simulink model "example"  (Simulink 7.0)
settings: Solver=ode4  StartTime=0.0  StopTime=100  FixedStep=0.01  RelTol=1e-3
values from neighbouring files (symbols this model uses):
  TID = min('TI' == AFT(1:2))    [PAS_callback.m]    (also in PSTID_callback.m = [block '/TID'])
libraries: simulink x280
(part 1 of 15)
settings Model: Creator=jza  LastModifiedBy=jza

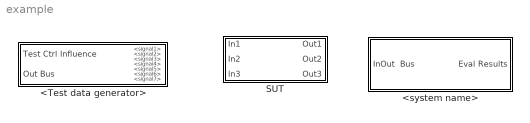
== system example ==
  <Test data generator> : Subsystem  mask{No=4, So=7, T=off}
      mask prompts: No "Number of Requirements"; So "Number of Signals"; T "Do you want to shut off the mask"
      mask StyleString: popup(1|2|3|4|5|6|7|8|9|10|11|12|13|14|15|16|17|18|19|20),popup(1|2|3|4|5|6|7|8|9|10|11|12|13|14|15|16|17|18|19|20),checkbox
      mask CallbackString: Test_D_Gen(gcb);|Test_D_Gen_S(gcb,-1);|shut_mask(gcb);
  <system name> : Subsystem  Description=Test evaluation system template. Create a new test evaluation system from this template.  mask{No=5, T=off}
      mask prompts: No "Number of Requirements"; T "Shut off the mask"
      mask StyleString: popup(1|2|3|4|5|6|7|8|9|10|11|12|13|14|15|16|17|18|19|20),checkbox
      mask CallbackString: system_name2(gcb);|shut_mask(gcb);
  SUT : Subsystem

== system example/<Test data generator> ==
  Test Ctrl Influence : Inport  OutDataType=sfix(16)  OutScaling=2^0
  Out Bus : Inport  Port=2  OutDataType=sfix(16)  OutScaling=2^0
  <Requirement name> : Subsystem
  <Requirement name>2 : Subsystem
  <Requirement name>3 : Subsystem
  <Requirement name>4 : Subsystem
  switch <signal1> : MultiPortSwitch  zeroidx=on
  switch <signal2> : MultiPortSwitch  zeroidx=on
  switch <signal3> : MultiPortSwitch  zeroidx=on
  switch <signal4> : MultiPortSwitch  zeroidx=on
  switch <signal5> : MultiPortSwitch  zeroidx=on
  switch <signal6> : MultiPortSwitch  zeroidx=on
  switch <signal7> : MultiPortSwitch  zeroidx=on
  <signal1> : Outport  OutDataType=sfix(16)  OutScaling=2^0
  <signal2> : Outport  Port=2  OutDataType=sfix(16)  OutScaling=2^0
  <signal3> : Outport  Port=3  OutDataType=sfix(16)  OutScaling=2^0
  <signal4> : Outport  Port=4  OutDataType=sfix(16)  OutScaling=2^0
  <signal5> : Outport  Port=5  OutDataType=sfix(16)  OutScaling=2^0
  <signal6> : Outport  Port=6  OutDataType=sfix(16)  OutScaling=2^0
  <signal7> : Outport  Port=7  OutDataType=sfix(16)  OutScaling=2^0
  wires:
  <Requirement name>/1(<signal1>) -> switch <signal1>/2
  switch <signal1>/1 -> <signal1>/1
  Out Bus/1 -> <Requirement name>/1(Out Bus), <Requirement name>2/1(Out Bus), <Requirement name>3/1(Out Bus), <Requirement name>4/1(Out Bus)
  Test Ctrl Influence/1 -> switch <signal1>/1, switch <signal2>/1, switch <signal3>/1, switch <signal4>/1, switch <signal5>/1, switch <signal6>/1, switch <signal7>/1
  <Requirement name>2/1(<signal1>) -> switch <signal1>/3
  <Requirement name>3/1(<signal1>) -> switch <signal1>/4
  <Requirement name>4/1(<signal1>) -> switch <signal1>/5
  switch <signal2>/1 -> <signal2>/1
  <Requirement name>/2(<signal2>) -> switch <signal2>/2
  <Requirement name>2/2(<signal2>) -> switch <signal2>/3
  <Requirement name>3/2(<signal2>) -> switch <signal2>/4
  <Requirement name>4/2(<signal2>) -> switch <signal2>/5
  switch <signal3>/1 -> <signal3>/1
  <Requirement name>/3(<signal3>) -> switch <signal3>/2
  <Requirement name>2/3(<signal3>) -> switch <signal3>/3
  <Requirement name>3/3(<signal3>) -> switch <signal3>/4
  <Requirement name>4/3(<signal3>) -> switch <signal3>/5
  switch <signal4>/1 -> <signal4>/1
  <Requirement name>/4(<signal4>) -> switch <signal4>/2
  <Requirement name>2/4(<signal4>) -> switch <signal4>/3
  <Requirement name>3/4(<signal4>) -> switch <signal4>/4
  <Requirement name>4/4(<signal4>) -> switch <signal4>/5
  switch <signal5>/1 -> <signal5>/1
  <Requirement name>/5(<signal5>) -> switch <signal5>/2
  <Requirement name>2/5(<signal5>) -> switch <signal5>/3
  <Requirement name>3/5(<signal5>) -> switch <signal5>/4
  <Requirement name>4/5(<signal5>) -> switch <signal5>/5
  switch <signal6>/1 -> <signal6>/1
  <Requirement name>/6(<signal6>) -> switch <signal6>/2
  <Requirement name>2/6(<signal6>) -> switch <signal6>/3
  <Requirement name>3/6(<signal6>) -> switch <signal6>/4
  <Requirement name>4/6(<signal6>) -> switch <signal6>/5
  switch <signal7>/1 -> <signal7>/1
  <Requirement name>/7(<signal7>) -> switch <signal7>/2
  <Requirement name>2/7(<signal7>) -> switch <signal7>/3
  <Requirement name>3/7(<signal7>) -> switch <signal7>/4
  <Requirement name>4/7(<signal7>) -> switch <signal7>/5

== system example/<system name> ==
  InOut  Bus : Inport  OutDataType=sfix(16)  OutScaling=2^0
  <Requirement name> : Subsystem  Description=Requirement template. Create a new requirement from this template.  mask{No=6}
      mask prompts: No "Number of single Validation Functions"
      mask StyleString: popup(1|2|3|4|5|6|7|8|9|10|11|12|13|14|15|16|17|18|19|20)
      mask CallbackString: ReqName_callback(gcb);
  <Requirement name>2 : Subsystem  Description=Requirement template. Create a new requirement from this template.  mask{No=1}
      mask prompts: No "Number of single Validation Functions"
      mask StyleString: popup(1|2|3|4|5|6|7|8|9|10|11|12|13|14|15|16|17|18|19|20)
      mask CallbackString: ReqName_callback(gcb);
  <Requirement name>3 : Subsystem  Description=Requirement template. Create a new requirement from this template.  mask{No=1}
      mask prompts: No "Number of single Validation Functions"
      mask StyleString: popup(1|2|3|4|5|6|7|8|9|10|11|12|13|14|15|16|17|18|19|20)
      mask CallbackString: ReqName_callback(gcb);
  <Requirement name>4 : Subsystem  Description=Requirement template. Create a new requirement from this template.  mask{No=1}
      mask prompts: No "Number of single Validation Functions"
      mask StyleString: popup(1|2|3|4|5|6|7|8|9|10|11|12|13|14|15|16|17|18|19|20)
      mask CallbackString: ReqName_callback(gcb);
  <Requirement name>5 : Subsystem  Description=Requirement template. Create a new requirement from this template.  mask{No=1}
      mask prompts: No "Number of single Validation Functions"
      mask StyleString: popup(1|2|3|4|5|6|7|8|9|10|11|12|13|14|15|16|17|18|19|20)
      mask CallbackString: ReqName_callback(gcb);
  Arbitration : Subsystem
  Bus Creator : BusCreator  Inputs=5
  Bus Creator1 : BusCreator  Inputs=2
  Bus Creator4 : BusCreator  Inputs=10
  Bus Selector : BusSelector  OutputSignals=signal1.signal1.signal1,signal2.signal1.signal1,signal3.signal1.signal1,signal4.signal1.signal1,signal5.signal1.signal1,signal.signal2.signal1,signal.signal3.signal1,signal.signal4.signal1,signal.signal5.signal1,signal.signal6.signal1
  Signal Conversion : SignalConversion  ConversionOutput=Bus copy
  Terminator : Terminator
  Eval Results : Outport  OutDataType=sfix(16)  OutScaling=2^0
  wires:
  Bus Creator1/1 -> Eval Results/1
  Bus Creator4/1 -> Bus Creator1/2
  Signal Conversion/1 -> <Requirement name>/1(InOut Bus), <Requirement name>2/1(InOut Bus), <Requirement name>3/1(InOut Bus), <Requirement name>4/1(InOut Bus), <Requirement name>5/1(InOut Bus)
  Bus Creator/1 -> Terminator/1, Bus Selector/1
  InOut  Bus/1 -> Signal Conversion/1
  <Requirement name>/1(Test Info) -> Bus Creator/1
  Arbitration/1(Out1) -> Bus Creator1/1
  Bus Selector/1 -> Arbitration/1(In1), Bus Creator4/1  "<signal1>"
  <Requirement name>2/1(Test Info) -> Bus Creator/2
  Bus Selector/2 -> Bus Creator4/2, Arbitration/2(In2)  "<signal1>"
  <Requirement name>3/1(Test Info) -> Bus Creator/3
  Bus Selector/3 -> Bus Creator4/3, Arbitration/3(In3)  "<signal1>"
  <Requirement name>4/1(Test Info) -> Bus Creator/4
  Bus Selector/4 -> Bus Creator4/4, Arbitration/4(In4)  "<signal1>"
  <Requirement name>5/1(Test Info) -> Bus Creator/5
  Bus Selector/5 -> Bus Creator4/5, Arbitration/5(In5)  "<signal1>"
  Bus Selector/6 -> Arbitration/6(In6), Bus Creator4/6  "<signal1>"
  Bus Selector/7 -> Arbitration/7(In7), Bus Creator4/7  "<signal1>"
  Bus Selector/8 -> Arbitration/8(In8), Bus Creator4/8  "<signal1>"
  Bus Selector/9 -> Arbitration/9(In9), Bus Creator4/9  "<signal1>"
  Bus Selector/10 -> Arbitration/10(In10), Bus Creator4/10  "<signal1>"

== system example/SUT ==
  In1 : Inport  OutDataType=sfix(16)  OutScaling=2^0
  In2 : Inport  Port=2  OutDataType=sfix(16)  OutScaling=2^0
  In3 : Inport  Port=3  OutDataType=sfix(16)  OutScaling=2^0
  Out1 : Outport  OutDataType=sfix(16)  OutScaling=2^0
  Out2 : Outport  Port=2  OutDataType=sfix(16)  OutScaling=2^0
  Out3 : Outport  Port=3  OutDataType=sfix(16)  OutScaling=2^0
  wires:
  In1/1 -> Out1/1
  In2/1 -> Out2/1
  In3/1 -> Out3/1

== system example/<Test data generator>/<Requirement name> ==
  Out Bus : Inport  OutDataType=sfix(16)  OutScaling=2^0
  <Preconditions name> : Subsystem
  Initialisation & Stabilisation : Subsystem
  Sequencing of test data in time due to Preconditions : Stateflow chart
  switch <signal1> : MultiPortSwitch  Inputs=2
  switch <signal2> : MultiPortSwitch  Inputs=2
  switch <signal3> : MultiPortSwitch  Inputs=2
  switch <signal4> : MultiPortSwitch  Inputs=2
  switch <signal5> : MultiPortSwitch  Inputs=2
  switch <signal6> : MultiPortSwitch  Inputs=2
  switch <signal7> : MultiPortSwitch  Inputs=2
  <signal1> : Outport  OutDataType=sfix(16)  OutScaling=2^0
  <signal2> : Outport  Port=2  OutDataType=sfix(16)  OutScaling=2^0
  <signal3> : Outport  Port=3  OutDataType=sfix(16)  OutScaling=2^0
  <signal4> : Outport  Port=4  OutDataType=sfix(16)  OutScaling=2^0
  <signal5> : Outport  Port=5  OutDataType=sfix(16)  OutScaling=2^0
  <signal6> : Outport  Port=6  OutDataType=sfix(16)  OutScaling=2^0
  <signal7> : Outport  Port=7  OutDataType=sfix(16)  OutScaling=2^0
  wires:
  Out Bus/1 -> <Preconditions name>/1(Out Bus)
  switch <signal1>/1 -> <signal1>/1
  <Preconditions name>/1(Activate) -> Sequencing of test data in time due to Preconditions/1(Activate)
  Sequencing of test data in time due to Preconditions/1(TDPre) -> switch <signal1>/1, switch <signal2>/1, switch <signal3>/1, switch <signal4>/1, switch <signal5>/1, switch <signal6>/1, switch <signal7>/1
  <Preconditions name>/2(<signal1>) -> switch <signal1>/2
  Initialisation & Stabilisation/1(<signal1>) -> switch <signal1>/3, switch <signal2>/3, switch <signal3>/3, switch <signal4>/3, switch <signal5>/3, switch <signal6>/3, switch <signal7>/3
  switch <signal2>/1 -> <signal2>/1
  <Preconditions name>/3(<signal2>) -> switch <signal2>/2
  switch <signal3>/1 -> <signal3>/1
  <Preconditions name>/4(<signal3>) -> switch <signal3>/2
  switch <signal4>/1 -> <signal4>/1
  <Preconditions name>/5(<signal4>) -> switch <signal4>/2
  switch <signal5>/1 -> <signal5>/1
  <Preconditions name>/6(<signal5>) -> switch <signal5>/2
  switch <signal6>/1 -> <signal6>/1
  <Preconditions name>/7(<signal6>) -> switch <signal6>/2
  switch <signal7>/1 -> <signal7>/1
  <Preconditions name>/8(<signal7>) -> switch <signal7>/2

== system example/<Test data generator>/<Requirement name>2 ==
  Out Bus : Inport  OutDataType=sfix(16)  OutScaling=2^0
  <Preconditions name> : Subsystem
  Initialisation & Stabilisation : Subsystem
  Sequencing of test data in time due to Preconditions : Stateflow chart
  switch <signal1> : MultiPortSwitch  Inputs=2
  switch <signal2> : MultiPortSwitch  Inputs=2
  switch <signal3> : MultiPortSwitch  Inputs=2
  switch <signal4> : MultiPortSwitch  Inputs=2
  switch <signal5> : MultiPortSwitch  Inputs=2
  switch <signal6> : MultiPortSwitch  Inputs=2
  switch <signal7> : MultiPortSwitch  Inputs=2
  <signal1> : Outport  OutDataType=sfix(16)  OutScaling=2^0
  <signal2> : Outport  Port=2  OutDataType=sfix(16)  OutScaling=2^0
  <signal3> : Outport  Port=3  OutDataType=sfix(16)  OutScaling=2^0
  <signal4> : Outport  Port=4  OutDataType=sfix(16)  OutScaling=2^0
  <signal5> : Outport  Port=5  OutDataType=sfix(16)  OutScaling=2^0
  <signal6> : Outport  Port=6  OutDataType=sfix(16)  OutScaling=2^0
  <signal7> : Outport  Port=7  OutDataType=sfix(16)  OutScaling=2^0
  wires:
  Initialisation & Stabilisation/1(<signal1>) -> switch <signal1>/3, switch <signal2>/3, switch <signal3>/3, switch <signal4>/3, switch <signal5>/3, switch <signal6>/3, switch <signal7>/3
  <Preconditions name>/2(<signal1>) -> switch <signal1>/2
  Sequencing of test data in time due to Preconditions/1(TDPre) -> switch <signal1>/1, switch <signal2>/1, switch <signal3>/1, switch <signal4>/1, switch <signal5>/1, switch <signal6>/1, switch <signal7>/1
  <Preconditions name>/1(Activate) -> Sequencing of test data in time due to Preconditions/1(Activate)
  switch <signal1>/1 -> <signal1>/1
  Out Bus/1 -> <Preconditions name>/1(Out Bus)
  switch <signal2>/1 -> <signal2>/1
  <Preconditions name>/3(<signal2>) -> switch <signal2>/2
  switch <signal3>/1 -> <signal3>/1
  <Preconditions name>/4(<signal3>) -> switch <signal3>/2
  switch <signal4>/1 -> <signal4>/1
  <Preconditions name>/5(<signal4>) -> switch <signal4>/2
  switch <signal5>/1 -> <signal5>/1
  <Preconditions name>/6(<signal5>) -> switch <signal5>/2
  switch <signal6>/1 -> <signal6>/1
  <Preconditions name>/7(<signal6>) -> switch <signal6>/2
  switch <signal7>/1 -> <signal7>/1
  <Preconditions name>/8(<signal7>) -> switch <signal7>/2

== system example/<Test data generator>/<Requirement name>3 ==
  Out Bus : Inport  OutDataType=sfix(16)  OutScaling=2^0
  <Preconditions name> : Subsystem
  Initialisation & Stabilisation : Subsystem
  Sequencing of test data in time due to Preconditions : Stateflow chart
  switch <signal1> : MultiPortSwitch  Inputs=2
  switch <signal2> : MultiPortSwitch  Inputs=2
  switch <signal3> : MultiPortSwitch  Inputs=2
  switch <signal4> : MultiPortSwitch  Inputs=2
  switch <signal5> : MultiPortSwitch  Inputs=2
  switch <signal6> : MultiPortSwitch  Inputs=2
  switch <signal7> : MultiPortSwitch  Inputs=2
  <signal1> : Outport  OutDataType=sfix(16)  OutScaling=2^0
  <signal2> : Outport  Port=2  OutDataType=sfix(16)  OutScaling=2^0
  <signal3> : Outport  Port=3  OutDataType=sfix(16)  OutScaling=2^0
  <signal4> : Outport  Port=4  OutDataType=sfix(16)  OutScaling=2^0
  <signal5> : Outport  Port=5  OutDataType=sfix(16)  OutScaling=2^0
  <signal6> : Outport  Port=6  OutDataType=sfix(16)  OutScaling=2^0
  <signal7> : Outport  Port=7  OutDataType=sfix(16)  OutScaling=2^0
  wires:
  Out Bus/1 -> <Preconditions name>/1(Out Bus)
  switch <signal1>/1 -> <signal1>/1
  <Preconditions name>/1(Activate) -> Sequencing of test data in time due to Preconditions/1(Activate)
  Sequencing of test data in time due to Preconditions/1(TDPre) -> switch <signal1>/1, switch <signal2>/1, switch <signal3>/1, switch <signal4>/1, switch <signal5>/1, switch <signal6>/1, switch <signal7>/1
  <Preconditions name>/2(<signal1>) -> switch <signal1>/2
  Initialisation & Stabilisation/1(<signal1>) -> switch <signal1>/3, switch <signal2>/3, switch <signal3>/3, switch <signal4>/3, switch <signal5>/3, switch <signal6>/3, switch <signal7>/3
  switch <signal2>/1 -> <signal2>/1
  <Preconditions name>/3(<signal2>) -> switch <signal2>/2
  switch <signal3>/1 -> <signal3>/1
  <Preconditions name>/4(<signal3>) -> switch <signal3>/2
  switch <signal4>/1 -> <signal4>/1
  <Preconditions name>/5(<signal4>) -> switch <signal4>/2
  switch <signal5>/1 -> <signal5>/1
  <Preconditions name>/6(<signal5>) -> switch <signal5>/2
  switch <signal6>/1 -> <signal6>/1
  <Preconditions name>/7(<signal6>) -> switch <signal6>/2
  switch <signal7>/1 -> <signal7>/1
  <Preconditions name>/8(<signal7>) -> switch <signal7>/2

== system example/<Test data generator>/<Requirement name>4 ==
  Out Bus : Inport  OutDataType=sfix(16)  OutScaling=2^0
  <Preconditions name> : Subsystem
  Initialisation & Stabilisation : Subsystem
  Sequencing of test data in time due to Preconditions : Stateflow chart
  switch <signal1> : MultiPortSwitch  Inputs=2
  switch <signal2> : MultiPortSwitch  Inputs=2
  switch <signal3> : MultiPortSwitch  Inputs=2
  switch <signal4> : MultiPortSwitch  Inputs=2
  switch <signal5> : MultiPortSwitch  Inputs=2
  switch <signal6> : MultiPortSwitch  Inputs=2
  switch <signal7> : MultiPortSwitch  Inputs=2
  <signal1> : Outport  OutDataType=sfix(16)  OutScaling=2^0
  <signal2> : Outport  Port=2  OutDataType=sfix(16)  OutScaling=2^0
  <signal3> : Outport  Port=3  OutDataType=sfix(16)  OutScaling=2^0
  <signal4> : Outport  Port=4  OutDataType=sfix(16)  OutScaling=2^0
  <signal5> : Outport  Port=5  OutDataType=sfix(16)  OutScaling=2^0
  <signal6> : Outport  Port=6  OutDataType=sfix(16)  OutScaling=2^0
  <signal7> : Outport  Port=7  OutDataType=sfix(16)  OutScaling=2^0
  wires:
  Initialisation & Stabilisation/1(<signal1>) -> switch <signal1>/3, switch <signal2>/3, switch <signal3>/3, switch <signal4>/3, switch <signal5>/3, switch <signal6>/3, switch <signal7>/3
  <Preconditions name>/2(<signal1>) -> switch <signal1>/2
  Sequencing of test data in time due to Preconditions/1(TDPre) -> switch <signal1>/1, switch <signal2>/1, switch <signal3>/1, switch <signal4>/1, switch <signal5>/1, switch <signal6>/1, switch <signal7>/1
  <Preconditions name>/1(Activate) -> Sequencing of test data in time due to Preconditions/1(Activate)
  switch <signal1>/1 -> <signal1>/1
  Out Bus/1 -> <Preconditions name>/1(Out Bus)
  switch <signal2>/1 -> <signal2>/1
  <Preconditions name>/3(<signal2>) -> switch <signal2>/2
  switch <signal3>/1 -> <signal3>/1
  <Preconditions name>/4(<signal3>) -> switch <signal3>/2
  switch <signal4>/1 -> <signal4>/1
  <Preconditions name>/5(<signal4>) -> switch <signal4>/2
  switch <signal5>/1 -> <signal5>/1
  <Preconditions name>/6(<signal5>) -> switch <signal5>/2
  switch <signal6>/1 -> <signal6>/1
  <Preconditions name>/7(<signal6>) -> switch <signal6>/2
  switch <signal7>/1 -> <signal7>/1
  <Preconditions name>/8(<signal7>) -> switch <signal7>/2

== system example/<system name>/<Requirement name> ==
  InOut Bus : Inport  OutDataType=sfix(16)  OutScaling=2^0
  <Assertions name> : Subsystem  Description=Assertions template. Create a new assertions block from this template.
  <Assertions name>2 : Subsystem  Description=Assertions template. Create a new assertions block from this template.
  <Assertions name>3 : Subsystem  Description=Assertions template. Create a new assertions block from this template.
  <Assertions name>4 : Subsystem  Description=Assertions template. Create a new assertions block from this template.
  <Assertions name>5 : Subsystem  Description=Assertions template. Create a new assertions block from this template.
  <Assertions name>6 : Subsystem  Description=Assertions template. Create a new assertions block from this template.
  <Preconditions name> : Subsystem  Description=Preconditions template. Create new preconditions blocks using this template.
  <Preconditions name>2 : Subsystem  Description=Preconditions template. Create new preconditions blocks using this template.
  <Preconditions name>3 : Subsystem  Description=Preconditions template. Create new preconditions blocks using this template.
  <Preconditions name>4 : Subsystem  Description=Preconditions template. Create new preconditions blocks using this template.
  <Preconditions name>5 : Subsystem  Description=Preconditions template. Create new preconditions blocks using this template.
  <Preconditions name>6 : Subsystem  Description=Preconditions template. Create new preconditions blocks using this template.
  Bus Creator : BusCreator  Inputs=6
  Test Info : Outport  OutDataType=sfix(16)  OutScaling=2^0
  wires:
  <Preconditions name>/1(Activate) -> <Assertions name>/1(Precond)
  Bus Creator/1 -> Test Info/1
  <Assertions name>/1(VF info) -> Bus Creator/1
  InOut Bus/1 -> <Preconditions name>/1(InOut Bus), <Assertions name>/2(InOut Bus), <Assertions name>2/2(InOut Bus), <Preconditions name>2/1(InOut Bus), <Assertions name>3/2(InOut Bus), <Preconditions name>3/1(InOut Bus), <Assertions name>4/2(InOut Bus), <Preconditions name>4/1(InOut Bus), <Assertions name>5/2(InOut Bus), <Preconditions name>5/1(InOut Bus), <Assertions name>6/2(InOut Bus), <Preconditions name>6/1(InOut Bus)
  <Preconditions name>2/1(Activate) -> <Assertions name>2/1(Precond)
  <Assertions name>2/1(VF info) -> Bus Creator/2
  <Preconditions name>3/1(Activate) -> <Assertions name>3/1(Precond)
  <Assertions name>3/1(VF info) -> Bus Creator/3
  <Preconditions name>4/1(Activate) -> <Assertions name>4/1(Precond)
  <Assertions name>4/1(VF info) -> Bus Creator/4
  <Preconditions name>5/1(Activate) -> <Assertions name>5/1(Precond)
  <Assertions name>5/1(VF info) -> Bus Creator/5
  <Preconditions name>6/1(Activate) -> <Assertions name>6/1(Precond)
  <Assertions name>6/1(VF info) -> Bus Creator/6

== system example/<system name>/<Requirement name>2 ==
  InOut Bus : Inport  OutDataType=sfix(16)  OutScaling=2^0
  <Assertions name> : Subsystem  Description=Assertions template. Create a new assertions block from this template.
  <Preconditions name> : Subsystem  Description=Preconditions template. Create new preconditions blocks using this template.
  Bus Creator : BusCreator  Inputs=1
  Test Info : Outport  OutDataType=sfix(16)  OutScaling=2^0
  wires:
  <Preconditions name>/1(Activate) -> <Assertions name>/1(Precond)
  Bus Creator/1 -> Test Info/1
  <Assertions name>/1(VF info) -> Bus Creator/1
  InOut Bus/1 -> <Preconditions name>/1(InOut Bus), <Assertions name>/2(InOut Bus)

== system example/<system name>/<Requirement name>3 ==
  InOut Bus : Inport  OutDataType=sfix(16)  OutScaling=2^0
  <Assertions name> : Subsystem  Description=Assertions template. Create a new assertions block from this template.
  <Preconditions name> : Subsystem  Description=Preconditions template. Create new preconditions blocks using this template.
  Bus Creator : BusCreator  Inputs=1
  Test Info : Outport  OutDataType=sfix(16)  OutScaling=2^0
  wires:
  <Preconditions name>/1(Activate) -> <Assertions name>/1(Precond)
  Bus Creator/1 -> Test Info/1
  <Assertions name>/1(VF info) -> Bus Creator/1
  InOut Bus/1 -> <Preconditions name>/1(InOut Bus), <Assertions name>/2(InOut Bus)

== system example/<system name>/<Requirement name>4 ==
  InOut Bus : Inport  OutDataType=sfix(16)  OutScaling=2^0
  <Assertions name> : Subsystem  Description=Assertions template. Create a new assertions block from this template.
  <Preconditions name> : Subsystem  Description=Preconditions template. Create new preconditions blocks using this template.
  Bus Creator : BusCreator  Inputs=1
  Test Info : Outport  OutDataType=sfix(16)  OutScaling=2^0
  wires:
  <Preconditions name>/1(Activate) -> <Assertions name>/1(Precond)
  Bus Creator/1 -> Test Info/1
  <Assertions name>/1(VF info) -> Bus Creator/1
  InOut Bus/1 -> <Preconditions name>/1(InOut Bus), <Assertions name>/2(InOut Bus)

== system example/<system name>/<Requirement name>5 ==
  InOut Bus : Inport  OutDataType=sfix(16)  OutScaling=2^0
  <Assertions name> : Subsystem  Description=Assertions template. Create a new assertions block from this template.
  <Preconditions name> : Subsystem  Description=Preconditions template. Create new preconditions blocks using this template.
  Bus Creator : BusCreator  Inputs=1
  Test Info : Outport  OutDataType=sfix(16)  OutScaling=2^0
  wires:
  <Preconditions name>/1(Activate) -> <Assertions name>/1(Precond)
  Bus Creator/1 -> Test Info/1
  <Assertions name>/1(VF info) -> Bus Creator/1
  InOut Bus/1 -> <Preconditions name>/1(InOut Bus), <Assertions name>/2(InOut Bus)

== system example/<system name>/Arbitration ==
  In1 : Inport  OutDataType=sfix(16)  OutScaling=2^0
  In2 : Inport  Port=2  OutDataType=sfix(16)  OutScaling=2^0
  In3 : Inport  Port=3  OutDataType=sfix(16)  OutScaling=2^0
  In4 : Inport  Port=4  OutDataType=sfix(16)  OutScaling=2^0
  In5 : Inport  Port=5  OutDataType=sfix(16)  OutScaling=2^0
  In6 : Inport  Port=6  OutDataType=sfix(16)  OutScaling=2^0
  In7 : Inport  Port=7  OutDataType=sfix(16)  OutScaling=2^0
  In8 : Inport  Port=8  OutDataType=sfix(16)  OutScaling=2^0
  In9 : Inport  Port=9  OutDataType=sfix(16)  OutScaling=2^0
  In10 : Inport  Port=10  OutDataType=sfix(16)  OutScaling=2^0
  Collect Verdicts : MinMax  Inputs=11  OutDataType=sfix(16)  OutScaling=2^0
  Memory : Memory  Orientation=left  X0=2
  Out1 : Outport  OutDataType=sfix(16)  OutScaling=2^0
  wires:
  In1/1 -> Collect Verdicts/1
  Collect Verdicts/1 -> Out1/1, Memory/1
  In2/1 -> Collect Verdicts/2
  In3/1 -> Collect Verdicts/3
  In4/1 -> Collect Verdicts/4
  In5/1 -> Collect Verdicts/5
  In6/1 -> Collect Verdicts/6
  In7/1 -> Collect Verdicts/7
  In8/1 -> Collect Verdicts/8
  In9/1 -> Collect Verdicts/9
  Memory/1 -> Collect Verdicts/11
  In10/1 -> Collect Verdicts/10

== system example/<Test data generator>/<Requirement name>/<Preconditions name> ==
  Out Bus : Inport  OutDataType=sfix(16)  OutScaling=2^0
  <Check> : Subsystem
  Feature generation : Subsystem  TreatAsAtomicUnit=on  mask{Param=0}
      mask prompts: Param "Mask Parameter 1:"
  Feature generation2 : Subsystem  TreatAsAtomicUnit=on  mask{Param=0}
      mask prompts: Param "Mask Parameter 1:"
  Feature generation3 : Subsystem  TreatAsAtomicUnit=on  mask{Param=0}
      mask prompts: Param "Mask Parameter 1:"
  Feature generation4 : Subsystem  TreatAsAtomicUnit=on  mask{Param=0}
      mask prompts: Param "Mask Parameter 1:"
  Feature generation5 : Subsystem  TreatAsAtomicUnit=on  mask{Param=0}
      mask prompts: Param "Mask Parameter 1:"
  Feature generation6 : Subsystem  TreatAsAtomicUnit=on  mask{Param=0}
      mask prompts: Param "Mask Parameter 1:"
  Feature generation7 : Subsystem  TreatAsAtomicUnit=on  mask{Param=0}
      mask prompts: Param "Mask Parameter 1:"
  Activate : Outport  OutDataType=sfix(16)  OutScaling=2^0
  <signal1> : Outport  Port=2  OutDataType=sfix(16)  OutScaling=2^0
  <signal2> : Outport  Port=3  OutDataType=sfix(16)  OutScaling=2^0
  <signal3> : Outport  Port=4  OutDataType=sfix(16)  OutScaling=2^0
  <signal4> : Outport  Port=5  OutDataType=sfix(16)  OutScaling=2^0
  <signal5> : Outport  Port=6  OutDataType=sfix(16)  OutScaling=2^0
  <signal6> : Outport  Port=7  OutDataType=sfix(16)  OutScaling=2^0
  <signal7> : Outport  Port=8  OutDataType=sfix(16)  OutScaling=2^0
  wires:
  Out Bus/1 -> <Check>/1(Out Bus)
  Feature generation/1(<signal1>) -> <signal1>/1
  <Check>/1(A) -> Activate/1
  Feature generation2/1(<signal1>) -> <signal2>/1
  Feature generation3/1(<signal1>) -> <signal3>/1
  Feature generation4/1(<signal1>) -> <signal4>/1
  Feature generation5/1(<signal1>) -> <signal5>/1
  Feature generation6/1(<signal1>) -> <signal6>/1
  Feature generation7/1(<signal1>) -> <signal7>/1

== system example/<Test data generator>/<Requirement name>/Initialisation & Stabilisation ==
  <Feature generation> : Subsystem  TreatAsAtomicUnit=on  mask{Param=0}
      mask prompts: Param "Mask Parameter 1:"
  <signal1> : Outport  OutDataType=sfix(16)  OutScaling=2^0
  wires:
  <Feature generation>/1(<signal1>) -> <signal1>/1

== system example/<Test data generator>/<Requirement name>2/<Preconditions name> ==
  Out Bus : Inport  OutDataType=sfix(16)  OutScaling=2^0
  <Check> : Subsystem
  Feature generation : Subsystem  TreatAsAtomicUnit=on  mask{Param=0}
      mask prompts: Param "Mask Parameter 1:"
  Feature generation2 : Subsystem  TreatAsAtomicUnit=on  mask{Param=0}
      mask prompts: Param "Mask Parameter 1:"
  Feature generation3 : Subsystem  TreatAsAtomicUnit=on  mask{Param=0}
      mask prompts: Param "Mask Parameter 1:"
  Feature generation4 : Subsystem  TreatAsAtomicUnit=on  mask{Param=0}
      mask prompts: Param "Mask Parameter 1:"
  Feature generation5 : Subsystem  TreatAsAtomicUnit=on  mask{Param=0}
      mask prompts: Param "Mask Parameter 1:"
  Feature generation6 : Subsystem  TreatAsAtomicUnit=on  mask{Param=0}
      mask prompts: Param "Mask Parameter 1:"
  Feature generation7 : Subsystem  TreatAsAtomicUnit=on  mask{Param=0}
      mask prompts: Param "Mask Parameter 1:"
  Activate : Outport  OutDataType=sfix(16)  OutScaling=2^0
  <signal1> : Outport  Port=2  OutDataType=sfix(16)  OutScaling=2^0
  <signal2> : Outport  Port=3  OutDataType=sfix(16)  OutScaling=2^0
  <signal3> : Outport  Port=4  OutDataType=sfix(16)  OutScaling=2^0
  <signal4> : Outport  Port=5  OutDataType=sfix(16)  OutScaling=2^0
  <signal5> : Outport  Port=6  OutDataType=sfix(16)  OutScaling=2^0
  <signal6> : Outport  Port=7  OutDataType=sfix(16)  OutScaling=2^0
  <signal7> : Outport  Port=8  OutDataType=sfix(16)  OutScaling=2^0
  wires:
  <Check>/1(A) -> Activate/1
  Feature generation/1(<signal1>) -> <signal1>/1
  Out Bus/1 -> <Check>/1(Out Bus)
  Feature generation2/1(<signal1>) -> <signal2>/1
  Feature generation3/1(<signal1>) -> <signal3>/1
  Feature generation4/1(<signal1>) -> <signal4>/1
  Feature generation5/1(<signal1>) -> <signal5>/1
  Feature generation6/1(<signal1>) -> <signal6>/1
  Feature generation7/1(<signal1>) -> <signal7>/1

== system example/<Test data generator>/<Requirement name>2/Initialisation & Stabilisation ==
  <Feature generation> : Subsystem  TreatAsAtomicUnit=on  mask{Param=0}
      mask prompts: Param "Mask Parameter 1:"
  <signal1> : Outport  OutDataType=sfix(16)  OutScaling=2^0
  wires:
  <Feature generation>/1(<signal1>) -> <signal1>/1

== system example/<Test data generator>/<Requirement name>3/<Preconditions name> ==
  Out Bus : Inport  OutDataType=sfix(16)  OutScaling=2^0
  <Check> : Subsystem
  Feature generation : Subsystem  TreatAsAtomicUnit=on  mask{Param=0}
      mask prompts: Param "Mask Parameter 1:"
  Feature generation2 : Subsystem  TreatAsAtomicUnit=on  mask{Param=0}
      mask prompts: Param "Mask Parameter 1:"
  Feature generation3 : Subsystem  TreatAsAtomicUnit=on  mask{Param=0}
      mask prompts: Param "Mask Parameter 1:"
  Feature generation4 : Subsystem  TreatAsAtomicUnit=on  mask{Param=0}
      mask prompts: Param "Mask Parameter 1:"
  Feature generation5 : Subsystem  TreatAsAtomicUnit=on  mask{Param=0}
      mask prompts: Param "Mask Parameter 1:"
  Feature generation6 : Subsystem  TreatAsAtomicUnit=on  mask{Param=0}
      mask prompts: Param "Mask Parameter 1:"
  Feature generation7 : Subsystem  TreatAsAtomicUnit=on  mask{Param=0}
      mask prompts: Param "Mask Parameter 1:"
  Activate : Outport  OutDataType=sfix(16)  OutScaling=2^0
  <signal1> : Outport  Port=2  OutDataType=sfix(16)  OutScaling=2^0
  <signal2> : Outport  Port=3  OutDataType=sfix(16)  OutScaling=2^0
  <signal3> : Outport  Port=4  OutDataType=sfix(16)  OutScaling=2^0
  <signal4> : Outport  Port=5  OutDataType=sfix(16)  OutScaling=2^0
  <signal5> : Outport  Port=6  OutDataType=sfix(16)  OutScaling=2^0
  <signal6> : Outport  Port=7  OutDataType=sfix(16)  OutScaling=2^0
  <signal7> : Outport  Port=8  OutDataType=sfix(16)  OutScaling=2^0
  wires:
  Out Bus/1 -> <Check>/1(Out Bus)
  Feature generation/1(<signal1>) -> <signal1>/1
  <Check>/1(A) -> Activate/1
  Feature generation2/1(<signal1>) -> <signal2>/1
  Feature generation3/1(<signal1>) -> <signal3>/1
  Feature generation4/1(<signal1>) -> <signal4>/1
  Feature generation5/1(<signal1>) -> <signal5>/1
  Feature generation6/1(<signal1>) -> <signal6>/1
  Feature generation7/1(<signal1>) -> <signal7>/1

== system example/<Test data generator>/<Requirement name>3/Initialisation & Stabilisation ==
  <Feature generation> : Subsystem  TreatAsAtomicUnit=on  mask{Param=0}
      mask prompts: Param "Mask Parameter 1:"
  <signal1> : Outport  OutDataType=sfix(16)  OutScaling=2^0
  wires:
  <Feature generation>/1(<signal1>) -> <signal1>/1

== system example/<Test data generator>/<Requirement name>4/<Preconditions name> ==
  Out Bus : Inport  OutDataType=sfix(16)  OutScaling=2^0
  <Check> : Subsystem
  Feature generation : Subsystem  TreatAsAtomicUnit=on  mask{Param=0}
      mask prompts: Param "Mask Parameter 1:"
  Feature generation2 : Subsystem  TreatAsAtomicUnit=on  mask{Param=0}
      mask prompts: Param "Mask Parameter 1:"
  Feature generation3 : Subsystem  TreatAsAtomicUnit=on  mask{Param=0}
      mask prompts: Param "Mask Parameter 1:"
  Feature generation4 : Subsystem  TreatAsAtomicUnit=on  mask{Param=0}
      mask prompts: Param "Mask Parameter 1:"
  Feature generation5 : Subsystem  TreatAsAtomicUnit=on  mask{Param=0}
      mask prompts: Param "Mask Parameter 1:"
  Feature generation6 : Subsystem  TreatAsAtomicUnit=on  mask{Param=0}
      mask prompts: Param "Mask Parameter 1:"
  Feature generation7 : Subsystem  TreatAsAtomicUnit=on  mask{Param=0}
      mask prompts: Param "Mask Parameter 1:"
  Activate : Outport  OutDataType=sfix(16)  OutScaling=2^0
  <signal1> : Outport  Port=2  OutDataType=sfix(16)  OutScaling=2^0
  <signal2> : Outport  Port=3  OutDataType=sfix(16)  OutScaling=2^0
  <signal3> : Outport  Port=4  OutDataType=sfix(16)  OutScaling=2^0
  <signal4> : Outport  Port=5  OutDataType=sfix(16)  OutScaling=2^0
  <signal5> : Outport  Port=6  OutDataType=sfix(16)  OutScaling=2^0
  <signal6> : Outport  Port=7  OutDataType=sfix(16)  OutScaling=2^0
  <signal7> : Outport  Port=8  OutDataType=sfix(16)  OutScaling=2^0
  wires:
  <Check>/1(A) -> Activate/1
  Feature generation/1(<signal1>) -> <signal1>/1
  Out Bus/1 -> <Check>/1(Out Bus)
  Feature generation2/1(<signal1>) -> <signal2>/1
  Feature generation3/1(<signal1>) -> <signal3>/1
  Feature generation4/1(<signal1>) -> <signal4>/1
  Feature generation5/1(<signal1>) -> <signal5>/1
  Feature generation6/1(<signal1>) -> <signal6>/1
  Feature generation7/1(<signal1>) -> <signal7>/1

== system example/<Test data generator>/<Requirement name>4/Initialisation & Stabilisation ==
  <Feature generation> : Subsystem  TreatAsAtomicUnit=on  mask{Param=0}
      mask prompts: Param "Mask Parameter 1:"
  <signal1> : Outport  OutDataType=sfix(16)  OutScaling=2^0
  wires:
  <Feature generation>/1(<signal1>) -> <signal1>/1

== system example/<system name>/<Requirement name>/<Assertions name> ==
  Precond : Inport  OutDataType=sfix(16)  OutScaling=2^0
  InOut Bus : Inport  Port=2  OutDataType=sfix(16)  OutScaling=2^0
  <Reference name> : Constant  OutDataType=sfix(16)  OutScaling=2^0
  Bus Creator : BusCreator  Inputs=1
  Bus Selector : BusSelector  OutputSignals=signal1
  Feature extraction : Subsystem  TreatAsAtomicUnit=on  mask{Param=0}
      mask prompts: Param "Mask Parameter 1:"
  PAS : Subsystem  mask{AFT=TID, AFD=600}
      mask prompts: AFT "Assertion feature type:"; AFD "Assertion feature delay (in time steps)"
      mask init:
      | PAS_init(gcb);
      mask StyleString: popup(TI|TDD|TID),edit
      mask CallbackString: PAS_callback(gcb);|
  Signal comparison : Subsystem  TreatAsAtomicUnit=on  mask{Param=0}
      mask prompts: Param "Mask Parameter 1:"
  VF info : Outport  OutDataType=sfix(16)  OutScaling=2^0
  wires:
  Bus Creator/1 -> VF info/1
  InOut Bus/1 -> Bus Selector/1
  Precond/1 -> PAS/1(Precond)
  PAS/1(VF Info) -> Bus Creator/1
  <Reference name>/1 -> Signal comparison/2(Ref)
  Feature extraction/3(A) -> Signal comparison/1(Sig)
  Feature extraction/2(T) -> PAS/3(T)
  Feature extraction/1(R) -> PAS/2(R)
  Bus Selector/1 -> Feature extraction/1(Sig)  "<signal1>"
  Signal comparison/1(V) -> PAS/4(V)

== system example/<system name>/<Requirement name>/<Assertions name>2 ==
  Precond : Inport  OutDataType=sfix(16)  OutScaling=2^0
  InOut Bus : Inport  Port=2  OutDataType=sfix(16)  OutScaling=2^0
  <Reference name> : Constant  OutDataType=sfix(16)  OutScaling=2^0
  Bus Creator : BusCreator  Inputs=1
  Bus Selector : BusSelector  OutputSignals=signal1
  Feature extraction : Subsystem  TreatAsAtomicUnit=on  mask{Param=0}
      mask prompts: Param "Mask Parameter 1:"
  PAS : Subsystem  mask{AFT=TID, AFD=600}
      mask prompts: AFT "Assertion feature type:"; AFD "Assertion feature delay (in time steps)"
      mask init:
      | PAS_init(gcb);
      mask StyleString: popup(TI|TDD|TID),edit
      mask CallbackString: PAS_callback(gcb);|
  Signal comparison : Subsystem  TreatAsAtomicUnit=on  mask{Param=0}
      mask prompts: Param "Mask Parameter 1:"
  VF info : Outport  OutDataType=sfix(16)  OutScaling=2^0
  wires:
  Bus Creator/1 -> VF info/1
  InOut Bus/1 -> Bus Selector/1
  Precond/1 -> PAS/1(Precond)
  PAS/1(VF Info) -> Bus Creator/1
  <Reference name>/1 -> Signal comparison/2(Ref)
  Feature extraction/3(A) -> Signal comparison/1(Sig)
  Feature extraction/2(T) -> PAS/3(T)
  Feature extraction/1(R) -> PAS/2(R)
  Bus Selector/1 -> Feature extraction/1(Sig)  "<signal1>"
  Signal comparison/1(V) -> PAS/4(V)

== system example/<system name>/<Requirement name>/<Assertions name>3 ==
  Precond : Inport  OutDataType=sfix(16)  OutScaling=2^0
  InOut Bus : Inport  Port=2  OutDataType=sfix(16)  OutScaling=2^0
  <Reference name> : Constant  OutDataType=sfix(16)  OutScaling=2^0
  Bus Creator : BusCreator  Inputs=1
  Bus Selector : BusSelector  OutputSignals=signal1
  Feature extraction : Subsystem  TreatAsAtomicUnit=on  mask{Param=0}
      mask prompts: Param "Mask Parameter 1:"
  PAS : Subsystem  mask{AFT=TID, AFD=600}
      mask prompts: AFT "Assertion feature type:"; AFD "Assertion feature delay (in time steps)"
      mask init:
      | PAS_init(gcb);
      mask StyleString: popup(TI|TDD|TID),edit
      mask CallbackString: PAS_callback(gcb);|
  Signal comparison : Subsystem  TreatAsAtomicUnit=on  mask{Param=0}
      mask prompts: Param "Mask Parameter 1:"
  VF info : Outport  OutDataType=sfix(16)  OutScaling=2^0
  wires:
  Bus Creator/1 -> VF info/1
  InOut Bus/1 -> Bus Selector/1
  Precond/1 -> PAS/1(Precond)
  PAS/1(VF Info) -> Bus Creator/1
  <Reference name>/1 -> Signal comparison/2(Ref)
  Feature extraction/3(A) -> Signal comparison/1(Sig)
  Feature extraction/2(T) -> PAS/3(T)
  Feature extraction/1(R) -> PAS/2(R)
  Bus Selector/1 -> Feature extraction/1(Sig)  "<signal1>"
  Signal comparison/1(V) -> PAS/4(V)

== system example/<system name>/<Requirement name>/<Assertions name>4 ==
  Precond : Inport  OutDataType=sfix(16)  OutScaling=2^0
  InOut Bus : Inport  Port=2  OutDataType=sfix(16)  OutScaling=2^0
  <Reference name> : Constant  OutDataType=sfix(16)  OutScaling=2^0
  Bus Creator : BusCreator  Inputs=1
  Bus Selector : BusSelector  OutputSignals=signal1
  Feature extraction : Subsystem  TreatAsAtomicUnit=on  mask{Param=0}
      mask prompts: Param "Mask Parameter 1:"
  PAS : Subsystem  mask{AFT=TID, AFD=600}
      mask prompts: AFT "Assertion feature type:"; AFD "Assertion feature delay (in time steps)"
      mask init:
      | PAS_init(gcb);
      mask StyleString: popup(TI|TDD|TID),edit
      mask CallbackString: PAS_callback(gcb);|
  Signal comparison : Subsystem  TreatAsAtomicUnit=on  mask{Param=0}
      mask prompts: Param "Mask Parameter 1:"
  VF info : Outport  OutDataType=sfix(16)  OutScaling=2^0
  wires:
  Bus Creator/1 -> VF info/1
  InOut Bus/1 -> Bus Selector/1
  Precond/1 -> PAS/1(Precond)
  PAS/1(VF Info) -> Bus Creator/1
  <Reference name>/1 -> Signal comparison/2(Ref)
  Feature extraction/3(A) -> Signal comparison/1(Sig)
  Feature extraction/2(T) -> PAS/3(T)
  Feature extraction/1(R) -> PAS/2(R)
  Bus Selector/1 -> Feature extraction/1(Sig)  "<signal1>"
  Signal comparison/1(V) -> PAS/4(V)

== system example/<system name>/<Requirement name>/<Assertions name>5 ==
  Precond : Inport  OutDataType=sfix(16)  OutScaling=2^0
  InOut Bus : Inport  Port=2  OutDataType=sfix(16)  OutScaling=2^0
  <Reference name> : Constant  OutDataType=sfix(16)  OutScaling=2^0
  Bus Creator : BusCreator  Inputs=1
  Bus Selector : BusSelector  OutputSignals=signal1
  Feature extraction : Subsystem  TreatAsAtomicUnit=on  mask{Param=0}
      mask prompts: Param "Mask Parameter 1:"
  PAS : Subsystem  mask{AFT=TID, AFD=600}
      mask prompts: AFT "Assertion feature type:"; AFD "Assertion feature delay (in time steps)"
      mask init:
      | PAS_init(gcb);
      mask StyleString: popup(TI|TDD|TID),edit
      mask CallbackString: PAS_callback(gcb);|
  Signal comparison : Subsystem  TreatAsAtomicUnit=on  mask{Param=0}
      mask prompts: Param "Mask Parameter 1:"
  VF info : Outport  OutDataType=sfix(16)  OutScaling=2^0
  wires:
  Bus Creator/1 -> VF info/1
  InOut Bus/1 -> Bus Selector/1
  Precond/1 -> PAS/1(Precond)
  PAS/1(VF Info) -> Bus Creator/1
  <Reference name>/1 -> Signal comparison/2(Ref)
  Feature extraction/3(A) -> Signal comparison/1(Sig)
  Feature extraction/2(T) -> PAS/3(T)
  Feature extraction/1(R) -> PAS/2(R)
  Bus Selector/1 -> Feature extraction/1(Sig)  "<signal1>"
  Signal comparison/1(V) -> PAS/4(V)

== system example/<system name>/<Requirement name>/<Assertions name>6 ==
  Precond : Inport  OutDataType=sfix(16)  OutScaling=2^0
  InOut Bus : Inport  Port=2  OutDataType=sfix(16)  OutScaling=2^0
  <Reference name> : Constant  OutDataType=sfix(16)  OutScaling=2^0
  Bus Creator : BusCreator  Inputs=1
  Bus Selector : BusSelector  OutputSignals=signal1
  Feature extraction : Subsystem  TreatAsAtomicUnit=on  mask{Param=0}
      mask prompts: Param "Mask Parameter 1:"
  PAS : Subsystem  mask{AFT=TID, AFD=600}
      mask prompts: AFT "Assertion feature type:"; AFD "Assertion feature delay (in time steps)"
      mask init:
      | PAS_init(gcb);
      mask StyleString: popup(TI|TDD|TID),edit
      mask CallbackString: PAS_callback(gcb);|
  Signal comparison : Subsystem  TreatAsAtomicUnit=on  mask{Param=0}
      mask prompts: Param "Mask Parameter 1:"
  VF info : Outport  OutDataType=sfix(16)  OutScaling=2^0
  wires:
  Bus Creator/1 -> VF info/1
  InOut Bus/1 -> Bus Selector/1
  Precond/1 -> PAS/1(Precond)
  PAS/1(VF Info) -> Bus Creator/1
  <Reference name>/1 -> Signal comparison/2(Ref)
  Feature extraction/3(A) -> Signal comparison/1(Sig)
  Feature extraction/2(T) -> PAS/3(T)
  Feature extraction/1(R) -> PAS/2(R)
  Bus Selector/1 -> Feature extraction/1(Sig)  "<signal1>"
  Signal comparison/1(V) -> PAS/4(V)

== system example/<system name>/<Requirement name>/<Preconditions name> ==
  InOut Bus : Inport  OutDataType=sfix(16)  OutScaling=2^0
  <Reference name> : Constant  OutDataType=sfix(16)  OutScaling=2^0
  Bus Selector : BusSelector  OutputSignals=signal1
  Feature extraction : Subsystem  TreatAsAtomicUnit=on  mask{Param=0}
      mask prompts: Param "Mask Parameter 1:"
  PS : Subsystem  mask(Feature layer: preconditions synchronization){NoTI=0, NoTDD=0, NoTID=1, TIdel=[0], TDDdel=[0]}
      mask prompts: NoTI "Time-independent features identifiable with or without a delay (TI)"; NoTDD "Triggered features identifiable with determinate delay or without a delay (TDD)"; NoTID "Triggered features identifiable with indeterminate delay (TID)"; TIdel "Time-independent features delays (in time steps). E.g. [0 1 0] for 3 features"; TDDdel "Triggered features delays (in time steps). E.g. [0 0] for 2 features"
      mask help: Use this block for synchronizing the precondition features. For changing the block inputs, use the parameters below. The output must be used for assertions activation.
      mask init:
      | PS_init(gcb);
      mask StyleString: popup(0|1|2|3|4|5|6|7|8|9),popup(0|1|2|3|4|5|6|7|8|9),popup(0|1|2|3|4|5|6|7|8|9),edit,edit
      mask CallbackString:
      | PSTI_callback(gcb);|PSTDD_callback(gcb);|PSTID_callback(gcb);|NoTI = str2double(get_param(gcb,'NoTI'));
      | TIdel = str2num(get_param(gcb,'TIdel'));
      | if NoTI ~= length(TIdel) && NoTI ~= 0
      |     error(['The number of delays entered (' num2str(length(TIdel)) ') does not correspond to the above specified number of time-independent features (' num2str(NoTI) ').']);
      | end|NoTDD = str2double(get_param(gcb,'NoTDD'));
      | TDDdel = str2num(get_param(gcb,'TDDdel'));
      | if NoTDD ~= length(TDDdel) && NoTDD ~= 0
      |     error(['The number of delays entered (' num2str(length(TDDdel)) ') does not correspond to the above specified number of triggered features with constant delay (' num2str(NoTDD) ').']);
      | end
  Signal comparison : Subsystem  TreatAsAtomicUnit=on  mask{Param=0}
      mask prompts: Param "Mask Parameter 1:"
  Activate : Outport  OutDataType=sfix(16)  OutScaling=2^0
  wires:
  InOut Bus/1 -> Bus Selector/1
  PS/1(Precond) -> Activate/1
  Signal comparison/1(A) -> PS/3(A TID1)
  <Reference name>/1 -> Signal comparison/2(Ref)
  Feature extraction/3(A) -> Signal comparison/1(Sig)
  Feature extraction/2(T) -> PS/2(T TID1)
  Feature extraction/1(R) -> PS/1(R TID1)
  Bus Selector/1 -> Feature extraction/1(Sig)  "<signal1>"

== system example/<system name>/<Requirement name>/<Preconditions name>2 ==
  InOut Bus : Inport  OutDataType=sfix(16)  OutScaling=2^0
  <Reference name> : Constant  OutDataType=sfix(16)  OutScaling=2^0
  Bus Selector : BusSelector  OutputSignals=signal1
  Feature extraction : Subsystem  TreatAsAtomicUnit=on  mask{Param=0}
      mask prompts: Param "Mask Parameter 1:"
  PS : Subsystem  mask(Feature layer: preconditions synchronization){NoTI=0, NoTDD=0, NoTID=1, TIdel=[0], TDDdel=[0]}
      mask prompts: NoTI "Time-independent features identifiable with or without a delay (TI)"; NoTDD "Triggered features identifiable with determinate delay or without a delay (TDD)"; NoTID "Triggered features identifiable with indeterminate delay (TID)"; TIdel "Time-independent features delays (in time steps). E.g. [0 1 0] for 3 features"; TDDdel "Triggered features delays (in time steps). E.g. [0 0] for 2 features"
      mask help: Use this block for synchronizing the precondition features. For changing the block inputs, use the parameters below. The output must be used for assertions activation.
      mask init:
      | PS_init(gcb);
      mask StyleString: popup(0|1|2|3|4|5|6|7|8|9),popup(0|1|2|3|4|5|6|7|8|9),popup(0|1|2|3|4|5|6|7|8|9),edit,edit
      mask CallbackString:
      | PSTI_callback(gcb);|PSTDD_callback(gcb);|PSTID_callback(gcb);|NoTI = str2double(get_param(gcb,'NoTI'));
      | TIdel = str2num(get_param(gcb,'TIdel'));
      | if NoTI ~= length(TIdel) && NoTI ~= 0
      |     error(['The number of delays entered (' num2str(length(TIdel)) ') does not correspond to the above specified number of time-independent features (' num2str(NoTI) ').']);
      | end|NoTDD = str2double(get_param(gcb,'NoTDD'));
      | TDDdel = str2num(get_param(gcb,'TDDdel'));
      | if NoTDD ~= length(TDDdel) && NoTDD ~= 0
      |     error(['The number of delays entered (' num2str(length(TDDdel)) ') does not correspond to the above specified number of triggered features with constant delay (' num2str(NoTDD) ').']);
      | end
  Signal comparison : Subsystem  TreatAsAtomicUnit=on  mask{Param=0}
      mask prompts: Param "Mask Parameter 1:"
  Activate : Outport  OutDataType=sfix(16)  OutScaling=2^0
  wires:
  InOut Bus/1 -> Bus Selector/1
  PS/1(Precond) -> Activate/1
  Signal comparison/1(A) -> PS/3(A TID1)
  <Reference name>/1 -> Signal comparison/2(Ref)
  Feature extraction/3(A) -> Signal comparison/1(Sig)
  Feature extraction/2(T) -> PS/2(T TID1)
  Feature extraction/1(R) -> PS/1(R TID1)
  Bus Selector/1 -> Feature extraction/1(Sig)  "<signal1>"

== system example/<system name>/<Requirement name>/<Preconditions name>3 ==
  InOut Bus : Inport  OutDataType=sfix(16)  OutScaling=2^0
  <Reference name> : Constant  OutDataType=sfix(16)  OutScaling=2^0
  Bus Selector : BusSelector  OutputSignals=signal1
  Feature extraction : Subsystem  TreatAsAtomicUnit=on  mask{Param=0}
      mask prompts: Param "Mask Parameter 1:"
  PS : Subsystem  mask(Feature layer: preconditions synchronization){NoTI=0, NoTDD=0, NoTID=1, TIdel=[0], TDDdel=[0]}
      mask prompts: NoTI "Time-independent features identifiable with or without a delay (TI)"; NoTDD "Triggered features identifiable with determinate delay or without a delay (TDD)"; NoTID "Triggered features identifiable with indeterminate delay (TID)"; TIdel "Time-independent features delays (in time steps). E.g. [0 1 0] for 3 features"; TDDdel "Triggered features delays (in time steps). E.g. [0 0] for 2 features"
      mask help: Use this block for synchronizing the precondition features. For changing the block inputs, use the parameters below. The output must be used for assertions activation.
      mask init:
      | PS_init(gcb);
      mask StyleString: popup(0|1|2|3|4|5|6|7|8|9),popup(0|1|2|3|4|5|6|7|8|9),popup(0|1|2|3|4|5|6|7|8|9),edit,edit
      mask CallbackString:
      | PSTI_callback(gcb);|PSTDD_callback(gcb);|PSTID_callback(gcb);|NoTI = str2double(get_param(gcb,'NoTI'));
      | TIdel = str2num(get_param(gcb,'TIdel'));
      | if NoTI ~= length(TIdel) && NoTI ~= 0
      |     error(['The number of delays entered (' num2str(length(TIdel)) ') does not correspond to the above specified number of time-independent features (' num2str(NoTI) ').']);
      | end|NoTDD = str2double(get_param(gcb,'NoTDD'));
      | TDDdel = str2num(get_param(gcb,'TDDdel'));
      | if NoTDD ~= length(TDDdel) && NoTDD ~= 0
      |     error(['The number of delays entered (' num2str(length(TDDdel)) ') does not correspond to the above specified number of triggered features with constant delay (' num2str(NoTDD) ').']);
      | end
  Signal comparison : Subsystem  TreatAsAtomicUnit=on  mask{Param=0}
      mask prompts: Param "Mask Parameter 1:"
  Activate : Outport  OutDataType=sfix(16)  OutScaling=2^0
  wires:
  InOut Bus/1 -> Bus Selector/1
  PS/1(Precond) -> Activate/1
  Signal comparison/1(A) -> PS/3(A TID1)
  <Reference name>/1 -> Signal comparison/2(Ref)
  Feature extraction/3(A) -> Signal comparison/1(Sig)
  Feature extraction/2(T) -> PS/2(T TID1)
  Feature extraction/1(R) -> PS/1(R TID1)
  Bus Selector/1 -> Feature extraction/1(Sig)  "<signal1>"
